simulink model "general_SD_model"  (R2021b)
settings: Solver=ode45  StartTime=0.0  StopTime=tfinal  FixedStep=T  MaxStep=0.01  RelTol=1e-12  AbsTol=1e-12  EnableMultiTasking=on
values from neighbouring files (symbols this model uses):
  period = 30    [part_a.m]    (also in part_b.m = 20; part_c.m = 40; part_d.m = 50)
  position_amplitude = 0.03    [paramGen.m]    (also in part_a.m = 0.1; part_ab.m; part_b.m = 0.1; part_c.m)
  position_offset = 0.15    [paramGen.m]    (also in part_a.m; part_ab.m; part_b.m; part_c.m)
  T = 0.001    [paramGen.m]    (also in part_a.m; part_ab.m; part_b.m; part_c.m)
libraries: cstblocks x5
settings Model: Creator=cnielsen  LastModifiedBy=mluser
settings SolverCC: AutoScaleAbsTol=off  AlgebraicLoopSolver=TrustRegion
settings DataIOCC: SaveFormat=Array  SignalLoggingSaveFormat=ModelDataLogs  SaveOutput=off  SaveTime=off  ReturnWorkspaceOutputs=off  Refine=5
settings OptimizationCC: ExpressionDepthLimit=2147483647  LifeSpan=inf
settings DebuggingCC: UnderspecifiedInitializationDetection=Classic  MergeDetectMultiDrivingBlocksExec=none  SolverPrmCheckMsg=warning  FcnCallInpInsideContextMsg=warning  StateNameClashWarn=warning  SFUnexpectedBacktrackingDiag=warning  SFNoUnconditionalDefaultTransitionDiag=warning  SFExecutionAtInitializationDiag=none  SFMachineParentedDataDiag=warning  ArithmeticOperatorsInVariantConditions=warning
settings HardwareCC: ProdBitPerPointer=32  ProdBitPerSizeT=32  ProdBitPerPtrDiffT=32  ProdLargestAtomicFloat=None  ProdIntDivRoundTo=Undefined  ProdEndianess=Unspecified  ProdWordSize=32  ProdHWDeviceType=32-bit Generic
settings ModelReferenceCC: PropagateSignalLabelsOutOfModel=off
settings SFSimCC: SimUseLocalCustomCode=off  CustomCodeUndefinedFunction=UseInterfaceOnly
settings RTWCC: RTWUseLocalCustomCode=off
settings CodeAppCC: StateflowObjectComments=on
settings GRTTargetCC: TargetLangStandard=C89/C90 (ANSI)  CombineOutputUpdateFcns=off  GRTInterface=on
settings ConfigComp: CovMetricSettings=dw  CovSaveCumulativeToWorkspaceVar=on  CovSaveSingleToWorkspaceVar=on  CovExternalEMLEnable=off

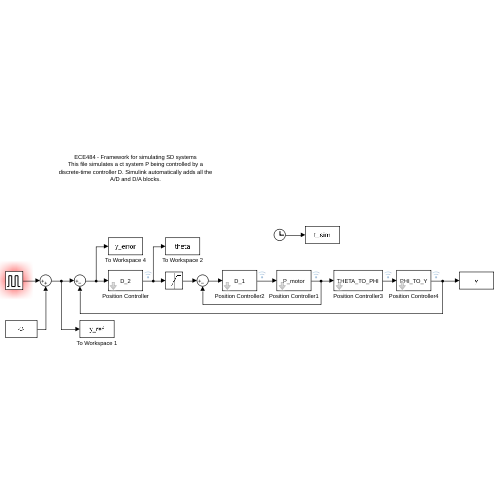
[thumbnail: Simulink's stored preview of the top-level diagram]
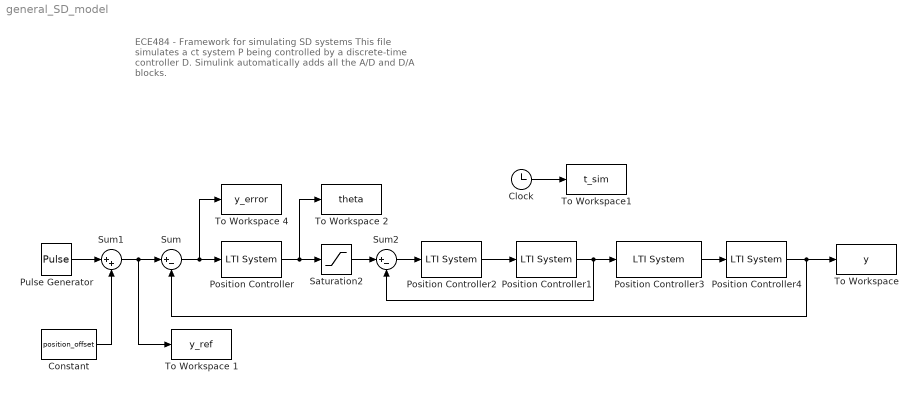
== system general_SD_model ==
  note: ECE484 - Framework for simulating SD systems
      | This file simulates a ct system P being controlled by a
      | discrete-time controller D. Simulink automatically adds all the
      | A/D and D/A blocks.
  Clock : Clock
  Constant : Constant  Value=position_offset
  Position Controller : cstblocks/LTI System  sys=D_2  IC=[]
  Position Controller1 : cstblocks/LTI System  sys=P_motor  IC=[]
  Position Controller2 : cstblocks/LTI System  sys=D_1  IC=[]
  Position Controller3 : cstblocks/LTI System  sys=THETA_TO_PHI  IC=[]
  Position Controller4 : cstblocks/LTI System  sys=PHI_TO_Y  IC=[]
  Pulse Generator : DiscretePulseGenerator  PulseType=Time based  Amplitude=position_amplitude  Period=period  PulseWidth=50  SampleTime=T
  Saturation2 : Saturate  UpperLimit=0.7  LowerLimit=-0.7
  Sum : Sum  Inputs=|+-
  Sum1 : Sum  Inputs=|++
  Sum2 : Sum  Inputs=|+-
  To Workspace : ToWorkspace  VariableName=y  SampleTime=T
  To Workspace 1 : ToWorkspace  VariableName=y_ref  SampleTime=T
  To Workspace 2 : ToWorkspace  VariableName=theta  SampleTime=T
  To Workspace 4 : ToWorkspace  VariableName=y_error  SampleTime=T
  To Workspace1 : ToWorkspace  VariableName=t_sim  SampleTime=T
  wires:
  Clock/1 -> To Workspace1/1
  Constant/1 -> Sum1/2
  Sum1/1 -> To Workspace 1/1, Sum/1
  Sum/1 -> Position Controller/1, To Workspace 4/1
  Position Controller/1 -> Saturation2/1, To Workspace 2/1
  Pulse Generator/1 -> Sum1/1
  Position Controller1/1 -> Position Controller3/1, Sum2/2
  Saturation2/1 -> Sum2/1
  Sum2/1 -> Position Controller2/1
  Position Controller2/1 -> Position Controller1/1
  Position Controller3/1 -> Position Controller4/1
  Position Controller4/1 -> Sum/2, To Workspace/1
